simulink model "ClosedLoop_V5_2020b"  (R2020b)
settings: Solver=ode4  StartTime=0.0  StopTime=TMax  FixedStep=DT  MaxStep=DT  RelTol=1e-3  EnableMultiTasking=on
undefined symbols (not defined in the file or in its folder): CertificationSettings, Control, DiscIntNeverNeededParam, Drivetrain, OutList, P_InitAngle, RPM_Init, sigbuilder_block, SimConfig, strmatch
libraries: simulink x11, simulink_extras x6
(part 2 of 3)

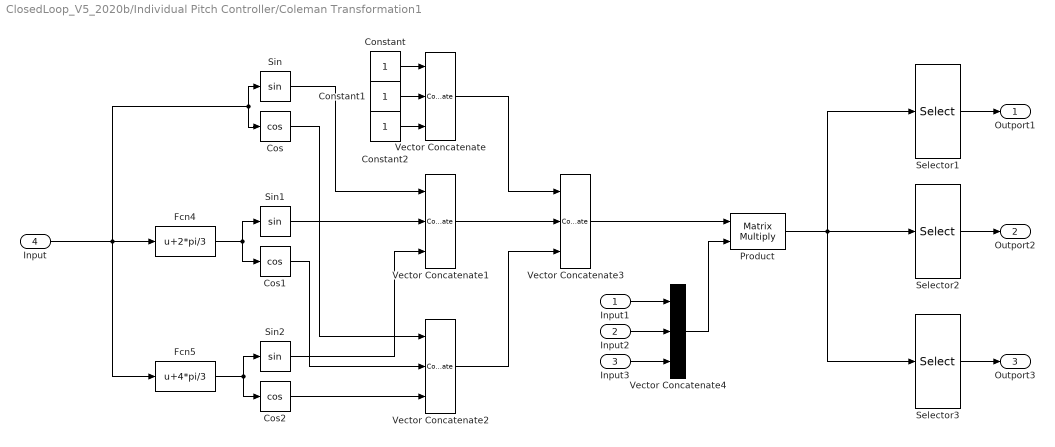
== system ClosedLoop_V5_2020b/Individual Pitch Controller/Coleman Transformation1 ==
  Input1 : Inport
  Input2 : Inport  Port=2
  Input3 : Inport  Port=3
  Input : Inport  Port=4
  Constant : Constant
  Constant1 : Constant
  Constant2 : Constant
  Cos : Trigonometry  Operator=cos
  Cos1 : Trigonometry  Operator=cos
  Cos2 : Trigonometry  Operator=cos
  Fcn4 : Fcn  Expr=u+2*pi/3
  Fcn5 : Fcn  Expr=u+4*pi/3
  Product : Product  Multiplication=Matrix(*)
  Selector1 : Selector  InputPortWidth=3  IndexOptions=Index vector (dialog)  Indices=[1]  OutputSizes=1
  Selector2 : Selector  InputPortWidth=3  IndexOptions=Index vector (dialog)  Indices=[2]  OutputSizes=1
  Selector3 : Selector  InputPortWidth=3  IndexOptions=Index vector (dialog)  Indices=[3]  OutputSizes=1
  Sin : Trigonometry
  Sin1 : Trigonometry
  Sin2 : Trigonometry
  Vector Concatenate{,1..2,4} (4 alike) : Concatenate  NumInputs=3
  Vector Concatenate3 : Concatenate  NumInputs=3  Mode=Multidimensional array  ConcatenateDimension=2
  Outport1 : Outport  VectorParamsAs1DForOutWhenUnconnected=off
  Outport2 : Outport  Port=2  VectorParamsAs1DForOutWhenUnconnected=off
  Outport3 : Outport  Port=3  VectorParamsAs1DForOutWhenUnconnected=off
  wires:
  Input3/1 -> Vector Concatenate4/3
  Input2/1 -> Vector Concatenate4/2
  Input1/1 -> Vector Concatenate4/1
  Constant2/1 -> Vector Concatenate/3
  Vector Concatenate3/1 -> Product/1
  Fcn4/1 -> Cos1/1, Sin1/1
  Vector Concatenate2/1 -> Vector Concatenate3/3
  Selector3/1 -> Outport3/1
  Selector2/1 -> Outport2/1
  Selector1/1 -> Outport1/1
  Vector Concatenate4/1 -> Product/2
  Vector Concatenate1/1 -> Vector Concatenate3/2
  Input/1 -> Cos/1, Sin/1, Fcn4/1, Fcn5/1
  Constant/1 -> Vector Concatenate/1
  Constant1/1 -> Vector Concatenate/2
  Sin2/1 -> Vector Concatenate1/3
  Cos1/1 -> Vector Concatenate2/2
  Cos/1 -> Vector Concatenate2/1
  Sin1/1 -> Vector Concatenate1/2
  Cos2/1 -> Vector Concatenate2/3
  Sin/1 -> Vector Concatenate1/1
  Product/1 -> Selector1/1, Selector2/1, Selector3/1
  Vector Concatenate/1 -> Vector Concatenate3/1
  Fcn5/1 -> Cos2/1, Sin2/1

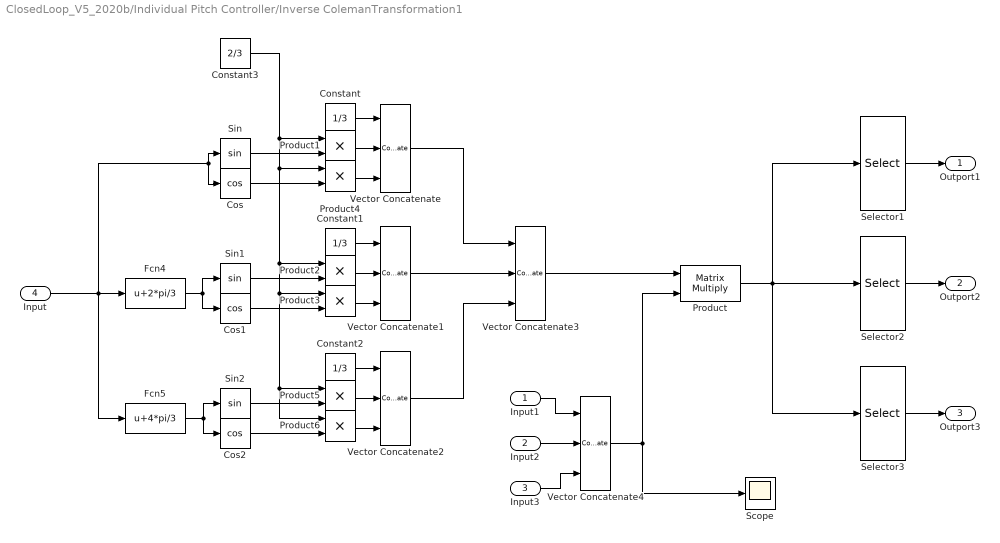
== system ClosedLoop_V5_2020b/Individual Pitch Controller/Inverse ColemanTransformation1 ==
  Input1 : Inport
  Input2 : Inport  Port=2
  Input3 : Inport  Port=3
  Input : Inport  Port=4
  Constant : Constant  Value=1/3
  Constant1 : Constant  Value=1/3
  Constant2 : Constant  Value=1/3
  Constant3 : Constant  Value=2/3
  Cos : Trigonometry  Operator=cos
  Cos1 : Trigonometry  Operator=cos
  Cos2 : Trigonometry  Operator=cos
  Fcn4 : Fcn  Expr=u+2*pi/3
  Fcn5 : Fcn  Expr=u+4*pi/3
  Product : Product  Multiplication=Matrix(*)
  Product{1..6} (6 alike) : Product
  Scope : Scope
  Selector1 : Selector  InputPortWidth=3  IndexOptions=Index vector (dialog)  Indices=[1]  OutputSizes=1
  Selector2 : Selector  InputPortWidth=3  IndexOptions=Index vector (dialog)  Indices=[2]  OutputSizes=1
  Selector3 : Selector  InputPortWidth=3  IndexOptions=Index vector (dialog)  Indices=[3]  OutputSizes=1
  Sin : Trigonometry
  Sin1 : Trigonometry
  Sin2 : Trigonometry
  Vector Concatenate : Concatenate  NumInputs=3  Mode=Multidimensional array
  Vector Concatenate1 : Concatenate  NumInputs=3  Mode=Multidimensional array
  Vector Concatenate2 : Concatenate  NumInputs=3  Mode=Multidimensional array
  Vector Concatenate3 : Concatenate  NumInputs=3  Mode=Multidimensional array  ConcatenateDimension=2
  Vector Concatenate4 : Concatenate  NumInputs=3
  Outport1 : Outport  VectorParamsAs1DForOutWhenUnconnected=off
  Outport2 : Outport  Port=2  VectorParamsAs1DForOutWhenUnconnected=off
  Outport3 : Outport  Port=3  VectorParamsAs1DForOutWhenUnconnected=off
  wires:
  Selector2/1 -> Outport2/1
  Selector3/1 -> Outport3/1
  Product/1 -> Selector1/1, Selector2/1, Selector3/1
  Selector1/1 -> Outport1/1
  Product2/1 -> Vector Concatenate1/2
  Product1/1 -> Vector Concatenate/2
  Constant/1 -> Vector Concatenate/1
  Vector Concatenate1/1 -> Vector Concatenate3/2
  Vector Concatenate2/1 -> Vector Concatenate3/3
  Vector Concatenate/1 -> Vector Concatenate3/1
  Vector Concatenate3/1 -> Product/1
  Input/1 -> Fcn4/1, Fcn5/1, Cos/1, Sin/1
  Product4/1 -> Vector Concatenate/3
  Sin1/1 -> Product2/2
  Constant1/1 -> Vector Concatenate1/1
  Product6/1 -> Vector Concatenate2/3
  Constant2/1 -> Vector Concatenate2/1
  Product3/1 -> Vector Concatenate1/3
  Sin/1 -> Product1/2
  Product5/1 -> Vector Concatenate2/2
  Input3/1 -> Vector Concatenate4/3
  Vector Concatenate4/1 -> Product/2, Scope/1
  Input1/1 -> Vector Concatenate4/1
  Input2/1 -> Vector Concatenate4/2
  Constant3/1 -> Product4/1, Product2/1, Product6/1, Product5/1, Product3/1, Product1/1
  Cos/1 -> Product4/2
  Cos1/1 -> Product3/2
  Sin2/1 -> Product5/2
  Cos2/1 -> Product6/2
  Fcn4/1 -> Sin1/1, Cos1/1
  Fcn5/1 -> Sin2/1, Cos2/1

== system ClosedLoop_V5_2020b/Individual Pitch Controller/Subsystem ==
  M_N2 : Inport
  Derivative : Derivative
  Gain : Gain  Gain=SimConfig.controller.IPC.K_P
  Gain1 : Gain  Gain=SimConfig.controller.IPC.K_D
  Gain3 : Gain  Gain=SimConfig.controller.IPC.K_I
  Integrator : Integrator
  Scope : Scope  NumInputPorts=5
  Scope1 : Scope  NumInputPorts=2
  Scope2 : Scope  NumInputPorts=2
  Scope3 : Scope  NumInputPorts=2
  Sum : Sum  Inputs=+++
  Input2 : Outport  VectorParamsAs1DForOutWhenUnconnected=off
  wires:
  Sum/1 -> Scope/4, Input2/1
  M_N2/1 -> Gain/1, Scope2/2, Gain3/1, Scope/5, Gain1/1  "E"
  Gain/1 -> Scope2/1, Scope/2, Sum/2  "P"
  Integrator/1 -> Scope1/2, Scope/3, Sum/3  "I"
  Derivative/1 -> Sum/1, Scope/1, Scope3/1  "D"
  Gain3/1 -> Integrator/1, Scope1/1
  Gain1/1 -> Derivative/1, Scope3/2

== system ClosedLoop_V5_2020b/Individual Pitch Controller/Subsystem1 ==
  M_N3 : Inport
  Derivative : Derivative
  Gain : Gain  Gain=SimConfig.controller.IPC.K_P
  Gain1 : Gain  Gain=SimConfig.controller.IPC.K_D
  Gain3 : Gain  Gain=SimConfig.controller.IPC.K_I
  Integrator : Integrator
  Scope : Scope  NumInputPorts=3
  Scope1 : Scope  NumInputPorts=2
  Scope2 : Scope  NumInputPorts=2
  Scope3 : Scope  NumInputPorts=2
  Sum : Sum  Inputs=+++
  Input3 : Outport  VectorParamsAs1DForOutWhenUnconnected=off
  wires:
  Derivative/1 -> Sum/1, Scope/1, Scope3/1  "D"
  Integrator/1 -> Scope/3, Sum/3, Scope1/2  "I"
  Gain/1 -> Sum/2, Scope/2, Scope2/1  "P"
  M_N3/1 -> Gain1/1, Scope2/2, Gain/1, Gain3/1
  Sum/1 -> Input3/1
  Gain3/1 -> Integrator/1, Scope1/1
  Gain1/1 -> Derivative/1, Scope3/2

== system ClosedLoop_V5_2020b/Notch filter TEF1/Notch filter TEF 1 ==
  u : Inport
  Damping : Constant  Value=0.06
  Frequ : Constant  Value=0.4*2*pi
  Gain : Gain  Gain=2
  Integrator : Integrator
  Integrator1 : Integrator
  Notch Gain : Constant  Value=10
  Product{,1..3} (4 alike) : Product
  Sum : Sum  Inputs=|++
  Sum1 : Sum  Inputs=++|
  Sum2 : Sum  Inputs=-+|
  Sum3 : Sum  Inputs=+-
  y : Outport
  wires:
  Product/1 -> Sum/2
  Sum/1 -> Sum3/2, y/1, Sum2/1
  Integrator/1 -> Product/1
  Integrator1/1 -> Product2/1
  Sum3/1 -> Integrator1/1
  Product1/1 -> Gain/1
  Product2/1 -> Sum1/2
  u/1 -> Sum/1, Product3/1, Sum3/1
  Product3/1 -> Sum2/2
  Sum2/1 -> Product1/2
  Sum1/1 -> Integrator/1
  Notch Gain/1 -> Product3/2
  Damping/1 -> Product1/1
  Frequ/1 -> Product/2, Product2/2
  Gain/1 -> Sum1/1

== system ClosedLoop_V5_2020b/Notch filter TEF1/Notch filter TEF 2 ==
  u : Inport
  Damping : Constant  Value=0.04
  Frequ : Constant  Value=0.6*2*pi
  Gain : Gain  Gain=2
  Integrator : Integrator
  Integrator1 : Integrator
  Notch Gain : Constant  Value=10
  Product{,1..3} (4 alike) : Product
  Sum : Sum  Inputs=|++
  Sum1 : Sum  Inputs=++|
  Sum2 : Sum  Inputs=-+|
  Sum3 : Sum  Inputs=+-
  y : Outport
  wires:
  Gain/1 -> Sum1/1
  Frequ/1 -> Product2/2, Product/2
  Damping/1 -> Product1/1
  Notch Gain/1 -> Product3/2
  Sum1/1 -> Integrator/1
  Sum2/1 -> Product1/2
  Product3/1 -> Sum2/2
  u/1 -> Sum3/1, Product3/1, Sum/1
  Product2/1 -> Sum1/2
  Product1/1 -> Gain/1
  Sum3/1 -> Integrator1/1
  Integrator1/1 -> Product2/1
  Integrator/1 -> Product/1
  Sum/1 -> Sum2/1, y/1, Sum3/2
  Product/1 -> Sum/2

== system ClosedLoop_V5_2020b/Notch filter TEF2/Notch filter TEF 1 ==
  u : Inport
  Damping : Constant  Value=0.06
  Frequ : Constant  Value=0.4*2*pi
  Gain : Gain  Gain=2
  Integrator : Integrator
  Integrator1 : Integrator
  Notch Gain : Constant  Value=10
  Product{,1..3} (4 alike) : Product
  Sum : Sum  Inputs=|++
  Sum1 : Sum  Inputs=++|
  Sum2 : Sum  Inputs=-+|
  Sum3 : Sum  Inputs=+-
  y : Outport
  wires:
  Gain/1 -> Sum1/1
  Frequ/1 -> Product2/2, Product/2
  Damping/1 -> Product1/1
  Notch Gain/1 -> Product3/2
  Sum1/1 -> Integrator/1
  Sum2/1 -> Product1/2
  Product3/1 -> Sum2/2
  u/1 -> Sum3/1, Product3/1, Sum/1
  Product2/1 -> Sum1/2
  Product1/1 -> Gain/1
  Sum3/1 -> Integrator1/1
  Integrator1/1 -> Product2/1
  Integrator/1 -> Product/1
  Sum/1 -> Sum2/1, y/1, Sum3/2
  Product/1 -> Sum/2

== system ClosedLoop_V5_2020b/Notch filter TEF2/Notch filter TEF 2 ==
  u : Inport
  Damping : Constant  Value=0.04
  Frequ : Constant  Value=0.6*2*pi
  Gain : Gain  Gain=2
  Integrator : Integrator
  Integrator1 : Integrator
  Notch Gain : Constant  Value=10
  Product{,1..3} (4 alike) : Product
  Sum : Sum  Inputs=|++
  Sum1 : Sum  Inputs=++|
  Sum2 : Sum  Inputs=-+|
  Sum3 : Sum  Inputs=+-
  y : Outport
  wires:
  Product/1 -> Sum/2
  Sum/1 -> Sum3/2, y/1, Sum2/1
  Integrator/1 -> Product/1
  Integrator1/1 -> Product2/1
  Sum3/1 -> Integrator1/1
  Product1/1 -> Gain/1
  Product2/1 -> Sum1/2
  u/1 -> Sum/1, Product3/1, Sum3/1
  Product3/1 -> Sum2/2
  Sum2/1 -> Product1/2
  Sum1/1 -> Integrator/1
  Notch Gain/1 -> Product3/2
  Damping/1 -> Product1/1
  Frequ/1 -> Product/2, Product2/2
  Gain/1 -> Sum1/1

== system ClosedLoop_V5_2020b/Notch filter TEF4/Notch filter TEF 1 ==
  u : Inport
  Damping : Constant  Value=0.06
  Frequ : Constant  Value=0.4*2*pi
  Gain : Gain  Gain=2
  Integrator : Integrator
  Integrator1 : Integrator
  Notch Gain : Constant  Value=10
  Product{,1..3} (4 alike) : Product
  Sum : Sum  Inputs=|++
  Sum1 : Sum  Inputs=++|
  Sum2 : Sum  Inputs=-+|
  Sum3 : Sum  Inputs=+-
  y : Outport
  wires:
  Gain/1 -> Sum1/1
  Frequ/1 -> Product2/2, Product/2
  Damping/1 -> Product1/1
  Notch Gain/1 -> Product3/2
  Sum1/1 -> Integrator/1
  Sum2/1 -> Product1/2
  Product3/1 -> Sum2/2
  u/1 -> Sum3/1, Product3/1, Sum/1
  Product2/1 -> Sum1/2
  Product1/1 -> Gain/1
  Sum3/1 -> Integrator1/1
  Integrator1/1 -> Product2/1
  Integrator/1 -> Product/1
  Sum/1 -> Sum2/1, y/1, Sum3/2
  Product/1 -> Sum/2

== system ClosedLoop_V5_2020b/Notch filter TEF4/Notch filter TEF 2 ==
  u : Inport
  Damping : Constant  Value=0.04
  Frequ : Constant  Value=0.6*2*pi
  Gain : Gain  Gain=2
  Integrator : Integrator
  Integrator1 : Integrator
  Notch Gain : Constant  Value=10
  Product{,1..3} (4 alike) : Product
  Sum : Sum  Inputs=|++
  Sum1 : Sum  Inputs=++|
  Sum2 : Sum  Inputs=-+|
  Sum3 : Sum  Inputs=+-
  y : Outport
  wires:
  Product/1 -> Sum/2
  Sum/1 -> Sum3/2, y/1, Sum2/1
  Integrator/1 -> Product/1
  Integrator1/1 -> Product2/1
  Sum3/1 -> Integrator1/1
  Product1/1 -> Gain/1
  Product2/1 -> Sum1/2
  u/1 -> Sum/1, Product3/1, Sum3/1
  Product3/1 -> Sum2/2
  Sum2/1 -> Product1/2
  Sum1/1 -> Integrator/1
  Notch Gain/1 -> Product3/2
  Damping/1 -> Product1/1
  Frequ/1 -> Product/2, Product2/2
  Gain/1 -> Sum1/1

== system ClosedLoop_V5_2020b/Notch filter TEF5/Notch filter TEF 1 ==
  u : Inport
  Damping : Constant  Value=0.06
  Frequ : Constant  Value=0.4*2*pi
  Gain : Gain  Gain=2
  Integrator : Integrator
  Integrator1 : Integrator
  Notch Gain : Constant  Value=10
  Product{,1..3} (4 alike) : Product
  Sum : Sum  Inputs=|++
  Sum1 : Sum  Inputs=++|
  Sum2 : Sum  Inputs=-+|
  Sum3 : Sum  Inputs=+-
  y : Outport
  wires:
  Gain/1 -> Sum1/1
  Frequ/1 -> Product2/2, Product/2
  Damping/1 -> Product1/1
  Notch Gain/1 -> Product3/2
  Sum1/1 -> Integrator/1
  Sum2/1 -> Product1/2
  Product3/1 -> Sum2/2
  u/1 -> Sum3/1, Product3/1, Sum/1
  Product2/1 -> Sum1/2
  Product1/1 -> Gain/1
  Sum3/1 -> Integrator1/1
  Integrator1/1 -> Product2/1
  Integrator/1 -> Product/1
  Sum/1 -> Sum2/1, y/1, Sum3/2
  Product/1 -> Sum/2

== system ClosedLoop_V5_2020b/Notch filter TEF5/Notch filter TEF 2 ==
  u : Inport
  Damping : Constant  Value=0.04
  Frequ : Constant  Value=0.6*2*pi
  Gain : Gain  Gain=2
  Integrator : Integrator
  Integrator1 : Integrator
  Notch Gain : Constant  Value=10
  Product{,1..3} (4 alike) : Product
  Sum : Sum  Inputs=|++
  Sum1 : Sum  Inputs=++|
  Sum2 : Sum  Inputs=-+|
  Sum3 : Sum  Inputs=+-
  y : Outport
  wires:
  Product/1 -> Sum/2
  Sum/1 -> Sum3/2, y/1, Sum2/1
  Integrator/1 -> Product/1
  Integrator1/1 -> Product2/1
  Sum3/1 -> Integrator1/1
  Product1/1 -> Gain/1
  Product2/1 -> Sum1/2
  u/1 -> Sum/1, Product3/1, Sum3/1
  Product3/1 -> Sum2/2
  Sum2/1 -> Product1/2
  Sum1/1 -> Integrator/1
  Notch Gain/1 -> Product3/2
  Damping/1 -> Product1/1
  Frequ/1 -> Product/2, Product2/2
  Gain/1 -> Sum1/1

== system ClosedLoop_V5_2020b/Notch filter TEF6/Notch filter TEF 1 ==
  u : Inport
  Damping : Constant  Value=0.06
  Frequ : Constant  Value=0.4*2*pi
  Gain : Gain  Gain=2
  Integrator : Integrator
  Integrator1 : Integrator
  Notch Gain : Constant  Value=10
  Product{,1..3} (4 alike) : Product
  Sum : Sum  Inputs=|++
  Sum1 : Sum  Inputs=++|
  Sum2 : Sum  Inputs=-+|
  Sum3 : Sum  Inputs=+-
  y : Outport
  wires:
  Gain/1 -> Sum1/1
  Frequ/1 -> Product2/2, Product/2
  Damping/1 -> Product1/1
  Notch Gain/1 -> Product3/2
  Sum1/1 -> Integrator/1
  Sum2/1 -> Product1/2
  Product3/1 -> Sum2/2
  u/1 -> Sum3/1, Product3/1, Sum/1
  Product2/1 -> Sum1/2
  Product1/1 -> Gain/1
  Sum3/1 -> Integrator1/1
  Integrator1/1 -> Product2/1
  Integrator/1 -> Product/1
  Sum/1 -> Sum2/1, y/1, Sum3/2
  Product/1 -> Sum/2

== system ClosedLoop_V5_2020b/Notch filter TEF6/Notch filter TEF 2 ==
  u : Inport
  Damping : Constant  Value=0.04
  Frequ : Constant  Value=0.6*2*pi
  Gain : Gain  Gain=2
  Integrator : Integrator
  Integrator1 : Integrator
  Notch Gain : Constant  Value=10
  Product{,1..3} (4 alike) : Product
  Sum : Sum  Inputs=|++
  Sum1 : Sum  Inputs=++|
  Sum2 : Sum  Inputs=-+|
  Sum3 : Sum  Inputs=+-
  y : Outport
  wires:
  Product/1 -> Sum/2
  Sum/1 -> Sum3/2, y/1, Sum2/1
  Integrator/1 -> Product/1
  Integrator1/1 -> Product2/1
  Sum3/1 -> Integrator1/1
  Product1/1 -> Gain/1
  Product2/1 -> Sum1/2
  u/1 -> Sum/1, Product3/1, Sum3/1
  Product3/1 -> Sum2/2
  Sum2/1 -> Product1/2
  Sum1/1 -> Integrator/1
  Notch Gain/1 -> Product3/2
  Damping/1 -> Product1/1
  Frequ/1 -> Product/2, Product2/2
  Gain/1 -> Sum1/1

== system ClosedLoop_V5_2020b/Notch filter Test/Notch filter 2 ==
  u : Inport
  gain : Inport  Port=2
  damping : Inport  Port=3
  frequency : Inport  Port=4
  Gain : Gain  Gain=2
  Integrator : Integrator
  Integrator1 : Integrator
  Product{,1..3} (4 alike) : Product
  Sum : Sum  Inputs=|++
  Sum1 : Sum  Inputs=++|
  Sum2 : Sum  Inputs=-+|
  Sum3 : Sum  Inputs=+-
  y : Outport
  wires:
  Gain/1 -> Sum1/1
  frequency/1 -> Product2/2, Product/2
  damping/1 -> Product1/1
  gain/1 -> Product3/2
  Sum1/1 -> Integrator/1
  Sum2/1 -> Product1/2
  Product3/1 -> Sum2/2
  u/1 -> Sum3/1, Product3/1, Sum/1
  Product2/1 -> Sum1/2
  Product1/1 -> Gain/1
  Sum3/1 -> Integrator1/1
  Integrator1/1 -> Product2/1
  Integrator/1 -> Product/1
  Sum/1 -> Sum2/1, y/1, Sum3/2
  Product/1 -> Sum/2

== system ClosedLoop_V5_2020b/Notch filter Test/Notch filter 3 ==
  u : Inport
  gain : Inport  Port=2
  damping : Inport  Port=3
  frequency : Inport  Port=4
  Gain : Gain  Gain=2
  Integrator : Integrator
  Integrator1 : Integrator
  Product{,1..3} (4 alike) : Product
  Sum : Sum  Inputs=|++
  Sum1 : Sum  Inputs=++|
  Sum2 : Sum  Inputs=-+|
  Sum3 : Sum  Inputs=+-
  y : Outport
  wires:
  Product/1 -> Sum/2
  Sum/1 -> Sum3/2, y/1, Sum2/1
  Integrator/1 -> Product/1
  Integrator1/1 -> Product2/1
  Sum3/1 -> Integrator1/1
  Product1/1 -> Gain/1
  Product2/1 -> Sum1/2
  u/1 -> Sum/1, Product3/1, Sum3/1
  Product3/1 -> Sum2/2
  Sum2/1 -> Product1/2
  Sum1/1 -> Integrator/1
  gain/1 -> Product3/2
  damping/1 -> Product1/1
  frequency/1 -> Product/2, Product2/2
  Gain/1 -> Sum1/1

== system ClosedLoop_V5_2020b/Notch filter Test/Notch filter neu ==
  u : Inport
  gain : Inport  Port=2
  damping : Inport  Port=3
  frequency : Inport  Port=4
  Gain : Gain  Gain=2
  Integrator : Integrator
  Integrator1 : Integrator
  Product{,1..3} (4 alike) : Product
  Sum : Sum  Inputs=|++
  Sum1 : Sum  Inputs=++|
  Sum2 : Sum  Inputs=-+|
  Sum3 : Sum  Inputs=+-
  y : Outport
  wires:
  Product/1 -> Sum/2
  Sum/1 -> Sum3/2, y/1, Sum2/1
  Integrator/1 -> Product/1
  Integrator1/1 -> Product2/1
  Sum3/1 -> Integrator1/1
  Product1/1 -> Gain/1
  Product2/1 -> Sum1/2
  u/1 -> Sum/1, Product3/1, Sum3/1
  Product3/1 -> Sum2/2
  Sum2/1 -> Product1/2
  Sum1/1 -> Integrator/1
  gain/1 -> Product3/2
  damping/1 -> Product1/1
  frequency/1 -> Product/2, Product2/2
  Gain/1 -> Sum1/1

== system ClosedLoop_V5_2020b/Notch filter Test/Subsystem ==
  u : Inport
  Notch filter TEF 1 : Subsystem
  Notch filter TEF 2 : Subsystem
  Scope : Scope  NumInputPorts=4
  Sum : Sum  Inputs=|++
  y : Outport
  wires:
  u/1 -> Notch filter TEF 2/1(u), Scope/4, Notch filter TEF 1/1(u)
  Notch filter TEF 1/1(y) -> Scope/2, Sum/1
  Notch filter TEF 2/1(y) -> Sum/2, Scope/3
  Sum/1 -> Scope/1, y/1

== system ClosedLoop_V5_2020b/Plot aerodynamic Data/Plot Angle of Attack ==
  OutData : Inport
  Scope1 : Scope  NumInputPorts=9
  Scope10 : Scope  NumInputPorts=3
  Scope12 : Scope  NumInputPorts=3
  Scope16 : Scope  NumInputPorts=3
  extract Angle of Attack : Fcn  Expr=u(strmatch('B1N1Alpha',OutList))
  extract Angle of Attack1 : Fcn  Expr=u(strmatch('B1N2Alpha',OutList))
  extract Angle of Attack2 : Fcn  Expr=u(strmatch('B1N3Alpha',OutList))
  extract Angle of Attack3 : Fcn  Expr=u(strmatch('B1N4Alpha',OutList))
  extract Angle of Attack4 : Fcn  Expr=u(strmatch('B1N5Alpha',OutList))
  extract Angle of Attack5 : Fcn  Expr=u(strmatch('B1N6Alpha',OutList))
  extract Angle of Attack6 : Fcn  Expr=u(strmatch('B1N7Alpha',OutList))
  extract Angle of Attack7 : Fcn  Expr=u(strmatch('B1N8Alpha',OutList))
  extract Angle of Attack8 : Fcn  Expr=u(strmatch('B1N9Alpha',OutList))
  wires:
  OutData/1 -> extract Angle of Attack8/1, extract Angle of Attack7/1, extract Angle of Attack6/1, extract Angle of Attack5/1, extract Angle of Attack4/1, extract Angle of Attack3/1, extract Angle of Attack2/1, extract Angle of Attack1/1, extract Angle of Attack/1
  extract Angle of Attack7/1 -> Scope1/8, Scope16/2  "Angle of Attack (deg)"
  extract Angle of Attack4/1 -> Scope1/5, Scope12/2  "Angle of Attack (deg)"
  extract Angle of Attack8/1 -> Scope1/9, Scope16/3  "Angle of Attack (deg)"
  extract Angle of Attack6/1 -> Scope1/7, Scope16/1  "Angle of Attack (deg)"
  extract Angle of Attack1/1 -> Scope1/2, Scope10/2  "Angle of Attack (deg)"
  extract Angle of Attack3/1 -> Scope1/4, Scope12/1  "Angle of Attack (deg)"
  extract Angle of Attack5/1 -> Scope1/6, Scope12/3  "Angle of Attack (deg)"
  extract Angle of Attack/1 -> Scope1/1, Scope10/1  "Angle of Attack (deg)"
  extract Angle of Attack2/1 -> Scope1/3, Scope10/3  "Angle of Attack (deg)"

== system ClosedLoop_V5_2020b/Plot aerodynamic Data/Plot Cd ==
  OutData : Inport
  Scope1 : Scope  NumInputPorts=9
  extract Cd : Fcn  Expr=u(strmatch('B1N1Cd',OutList))
  extract Cd1 : Fcn  Expr=u(strmatch('B1N2Cd',OutList))
  extract Cd2 : Fcn  Expr=u(strmatch('B1N3Cd',OutList))
  extract Cd3 : Fcn  Expr=u(strmatch('B1N4Cd',OutList))
  extract Cd4 : Fcn  Expr=u(strmatch('B1N5Cd',OutList))
  extract Cd5 : Fcn  Expr=u(strmatch('B1N6Cd',OutList))
  extract Cd6 : Fcn  Expr=u(strmatch('B1N7Cd',OutList))
  extract Cd7 : Fcn  Expr=u(strmatch('B1N8Cd',OutList))
  extract Cd8 : Fcn  Expr=u(strmatch('B1N9Cd',OutList))
  wires:
  OutData/1 -> extract Cd4/1, extract Cd5/1, extract Cd6/1, extract Cd8/1, extract Cd7/1, extract Cd3/1, extract Cd2/1, extract Cd1/1, extract Cd/1
  extract Cd/1 -> Scope1/1  "Cd"
  extract Cd1/1 -> Scope1/2  "Cd"
  extract Cd3/1 -> Scope1/4  "Cd"
  extract Cd2/1 -> Scope1/3  "Cd"
  extract Cd4/1 -> Scope1/5  "Cd"
  extract Cd5/1 -> Scope1/6  "Cd"
  extract Cd6/1 -> Scope1/7  "Cd"
  extract Cd7/1 -> Scope1/8  "Cd"
  extract Cd8/1 -> Scope1/9  "Cd"

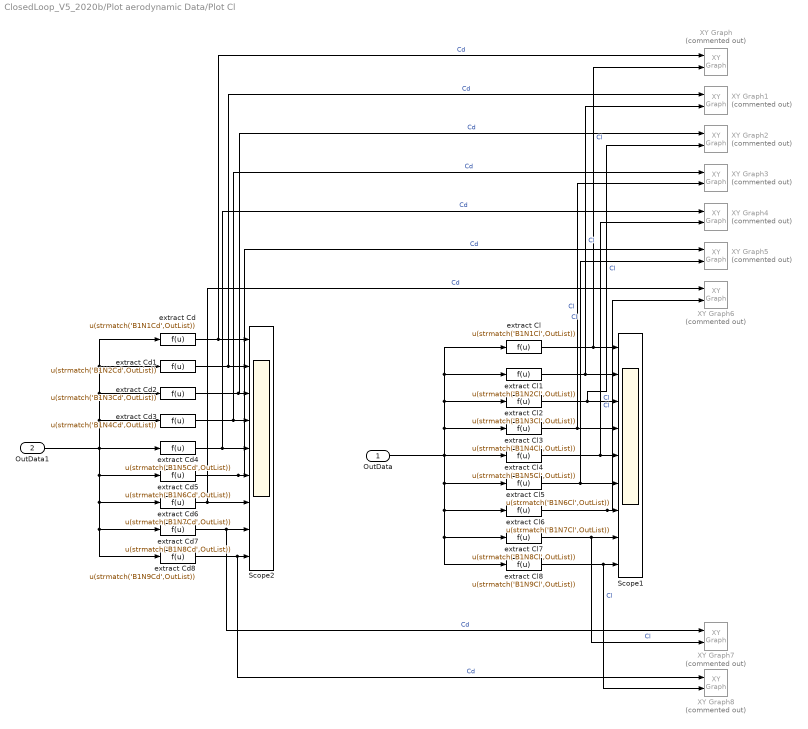
== system ClosedLoop_V5_2020b/Plot aerodynamic Data/Plot Cl ==
  OutData : Inport
  OutData1 : Inport  Port=2
  Scope1 : Scope  NumInputPorts=9
  Scope2 : Scope  NumInputPorts=9
  XY Graph{,1..8} (9 alike) : simulink/Sinks/XY Graph  Commented=on  xmin=-1  xmax=1  ymin=-1  ymax=1  st=-1
  extract Cd : Fcn  Expr=u(strmatch('B1N1Cd',OutList))
  extract Cd1 : Fcn  Expr=u(strmatch('B1N2Cd',OutList))
  extract Cd2 : Fcn  Expr=u(strmatch('B1N3Cd',OutList))
  extract Cd3 : Fcn  Expr=u(strmatch('B1N4Cd',OutList))
  extract Cd4 : Fcn  Expr=u(strmatch('B1N5Cd',OutList))
  extract Cd5 : Fcn  Expr=u(strmatch('B1N6Cd',OutList))
  extract Cd6 : Fcn  Expr=u(strmatch('B1N7Cd',OutList))
  extract Cd7 : Fcn  Expr=u(strmatch('B1N8Cd',OutList))
  extract Cd8 : Fcn  Expr=u(strmatch('B1N9Cd',OutList))
  extract Cl : Fcn  Expr=u(strmatch('B1N1Cl',OutList))
  extract Cl1 : Fcn  Expr=u(strmatch('B1N2Cl',OutList))
  extract Cl2 : Fcn  Expr=u(strmatch('B1N3Cl',OutList))
  extract Cl3 : Fcn  Expr=u(strmatch('B1N4Cl',OutList))
  extract Cl4 : Fcn  Expr=u(strmatch('B1N5Cl',OutList))
  extract Cl5 : Fcn  Expr=u(strmatch('B1N6Cl',OutList))
  extract Cl6 : Fcn  Expr=u(strmatch('B1N7Cl',OutList))
  extract Cl7 : Fcn  Expr=u(strmatch('B1N8Cl',OutList))
  extract Cl8 : Fcn  Expr=u(strmatch('B1N9Cl',OutList))
  wires:
  OutData/1 -> extract Cl/1, extract Cl1/1, extract Cl2/1, extract Cl3/1, extract Cl4/1, extract Cl5/1, extract Cl6/1, extract Cl8/1, extract Cl7/1
  extract Cl/1 -> XY Graph/2, Scope1/1  "Cl"
  extract Cl1/1 -> XY Graph1/2, Scope1/2  "Cl"
  extract Cl2/1 -> XY Graph2/2, Scope1/3  "Cl"
  extract Cl3/1 -> XY Graph3/2, Scope1/4  "Cl"
  extract Cl4/1 -> XY Graph4/2, Scope1/5  "Cl"
  extract Cl5/1 -> XY Graph5/2, Scope1/6  "Cl"
  extract Cl6/1 -> XY Graph6/2, Scope1/7  "Cl"
  extract Cl7/1 -> XY Graph7/2, Scope1/8  "Cl"
  extract Cl8/1 -> XY Graph8/2, Scope1/9  "Cl"
  extract Cd2/1 -> XY Graph2/1, Scope2/3  "Cd"
  extract Cd8/1 -> XY Graph8/1, Scope2/9  "Cd"
  extract Cd4/1 -> XY Graph4/1, Scope2/5  "Cd"
  extract Cd3/1 -> XY Graph3/1, Scope2/4  "Cd"
  extract Cd/1 -> XY Graph/1, Scope2/1  "Cd"
  OutData1/1 -> extract Cd4/1, extract Cd5/1, extract Cd6/1, extract Cd8/1, extract Cd7/1, extract Cd3/1, extract Cd2/1, extract Cd1/1, extract Cd/1
  extract Cd1/1 -> XY Graph1/1, Scope2/2  "Cd"
  extract Cd7/1 -> XY Graph7/1, Scope2/8  "Cd"
  extract Cd5/1 -> XY Graph5/1, Scope2/6  "Cd"
  extract Cd6/1 -> Scope2/7, XY Graph6/1  "Cd"

== system ClosedLoop_V5_2020b/Plot aerodynamic Data/Plot Pitch+Twist Angle ==
  OutData : Inport
  Add{,1..8} (9 alike) : Sum  Inputs=+-
  Scope1 : Scope  NumInputPorts=9
  Scope2 : Scope  NumInputPorts=9
  extract BldPitch1 (deg) : Fcn  Expr=u(strmatch('BldPitch1',OutList))
  extract Pitch+Twist angle : Fcn  Expr=u(strmatch('B1N1Theta',OutList))
  extract Pitch+Twist angle1 : Fcn  Expr=u(strmatch('B1N2Theta',OutList))
  extract Pitch+Twist angle2 : Fcn  Expr=u(strmatch('B1N3Theta',OutList))
  extract Pitch+Twist angle3 : Fcn  Expr=u(strmatch('B1N4Theta',OutList))
  extract Pitch+Twist angle4 : Fcn  Expr=u(strmatch('B1N5Theta',OutList))
  extract Pitch+Twist angle5 : Fcn  Expr=u(strmatch('B1N6Theta',OutList))
  extract Pitch+Twist angle6 : Fcn  Expr=u(strmatch('B1N7Theta',OutList))
  extract Pitch+Twist angle7 : Fcn  Expr=u(strmatch('B1N8Theta',OutList))
  extract Pitch+Twist angle8 : Fcn  Expr=u(strmatch('B1N9Theta',OutList))
  wires:
  extract Pitch+Twist angle/1 -> Add/1, Scope1/1  "Pitch+Twist angle (deg)"
  OutData/1 -> extract Pitch+Twist angle/1, extract Pitch+Twist angle1/1, extract Pitch+Twist angle2/1, extract Pitch+Twist angle3/1, extract Pitch+Twist angle4/1, extract Pitch+Twist angle5/1, extract Pitch+Twist angle6/1, extract BldPitch1 (deg)/1, extract Pitch+Twist angle8/1, extract Pitch+Twist angle7/1
  extract Pitch+Twist angle1/1 -> Add1/1, Scope1/2  "Pitch+Twist angle (deg)"
  extract Pitch+Twist angle2/1 -> Add2/1, Scope1/3  "Pitch+Twist angle (deg)"
  extract Pitch+Twist angle3/1 -> Add3/1, Scope1/4  "Pitch+Twist angle (deg)"
  extract Pitch+Twist angle4/1 -> Add4/1, Scope1/5  "Pitch+Twist angle (deg)"
  extract Pitch+Twist angle5/1 -> Add5/1, Scope1/6  "Pitch+Twist angle (deg)"
  extract Pitch+Twist angle6/1 -> Add6/1, Scope1/7  "Pitch+Twist angle (deg)"
  extract Pitch+Twist angle7/1 -> Add7/1, Scope1/8  "Pitch+Twist angle (deg)"
  extract Pitch+Twist angle8/1 -> Add8/1, Scope1/9  "Pitch+Twist angle (deg)"
  extract BldPitch1 (deg)/1 -> Add8/2, Add7/2, Add6/2, Add5/2, Add4/2, Add3/2, Add2/2, Add1/2, Add/2  "BldPitch1"
  Add/1 -> Scope2/1
  Add1/1 -> Scope2/2
  Add2/1 -> Scope2/3
  Add3/1 -> Scope2/4
  Add4/1 -> Scope2/5
  Add5/1 -> Scope2/6
  Add6/1 -> Scope2/7
  Add7/1 -> Scope2/8
  Add8/1 -> Scope2/9

== system ClosedLoop_V5_2020b/Plot aerodynamic Data/Plot Relative Wind Speed ==
  OutData1 : Inport
  Scope : Scope  NumInputPorts=9
  "extract Relative Wind Speed (m/s) at Blade 1, Node 1" : Fcn  Expr=u(strmatch('B1N1VRel',OutList))
  "extract Relative Wind Speed (m/s) at Blade 1, Node 2" : Fcn  Expr=u(strmatch('B1N2VRel',OutList))
  "extract Relative Wind Speed (m/s) at Blade 1, Node 3" : Fcn  Expr=u(strmatch('B1N3VRel',OutList))
  "extract Relative Wind Speed (m/s) at Blade 1, Node 4" : Fcn  Expr=u(strmatch('B1N4VRel',OutList))
  "extract Relative Wind Speed (m/s) at Blade 1, Node 5" : Fcn  Expr=u(strmatch('B1N5VRel',OutList))
  "extract Relative Wind Speed (m/s) at Blade 1, Node 6" : Fcn  Expr=u(strmatch('B1N6VRel',OutList))
  "extract Relative Wind Speed (m/s) at Blade 1, Node 7" : Fcn  Expr=u(strmatch('B1N7VRel',OutList))
  "extract Relative Wind Speed (m/s) at Blade 1, Node 8" : Fcn  Expr=u(strmatch('B1N8VRel',OutList))
  "extract Relative Wind Speed (m/s) at Blade 1, Node 9" : Fcn  Expr=u(strmatch('B1N9VRel',OutList))
  wires:
  OutData1/1 -> "extract Relative Wind Speed (m/s) at Blade 1, Node 9"/1, "extract Relative Wind Speed (m/s) at Blade 1, Node 8"/1, "extract Relative Wind Speed (m/s) at Blade 1, Node 7"/1, "extract Relative Wind Speed (m/s) at Blade 1, Node 6"/1, "extract Relative Wind Speed (m/s) at Blade 1, Node 5"/1, "extract Relative Wind Speed (m/s) at Blade 1, Node 4"/1, "extract Relative Wind Speed (m/s) at Blade 1, Node 3"/1, "extract Relative Wind Speed (m/s) at Blade 1, Node 2"/1, "extract Relative Wind Speed (m/s) at Blade 1, Node 1"/1
  "extract Relative Wind Speed (m/s) at Blade 1, Node 6"/1 -> Scope/6  "Relative Wind Speed (m/s) at Blade 1, Node 6"
  "extract Relative Wind Speed (m/s) at Blade 1, Node 7"/1 -> Scope/7  "Relative Wind Speed (m/s) at Blade 1, Node 7"
  "extract Relative Wind Speed (m/s) at Blade 1, Node 5"/1 -> Scope/5  "Relative Wind Speed (m/s) at Blade 1, Node 5"
  "extract Relative Wind Speed (m/s) at Blade 1, Node 9"/1 -> Scope/9  "Relative Wind Speed (m/s) at Blade 1, Node 9"
  "extract Relative Wind Speed (m/s) at Blade 1, Node 2"/1 -> Scope/2  "Relative Wind Speed (m/s) at Blade 1, Node 2"
  "extract Relative Wind Speed (m/s) at Blade 1, Node 1"/1 -> Scope/1  "Relative Wind Speed (m/s) at Blade 1, Node 1"
  "extract Relative Wind Speed (m/s) at Blade 1, Node 8"/1 -> Scope/8  "Relative Wind Speed (m/s) at Blade 1, Node 8"
  "extract Relative Wind Speed (m/s) at Blade 1, Node 4"/1 -> Scope/4  "Relative Wind Speed (m/s) at Blade 1, Node 4"
  "extract Relative Wind Speed (m/s) at Blade 1, Node 3"/1 -> Scope/3  "Relative Wind Speed (m/s) at Blade 1, Node 3"

== system ClosedLoop_V5_2020b/Plot aerodynamic Data/Plot Reynolds number ==
  note: B1N1Re      Reynolds number (in millions) at Blade 1, Node 1
      | B1N2Re      Reynolds number (in millions) at Blade 1, Node 2
      | B1N3Re      Reynolds number (in millions) at Blade 1, Node 3
      | B1N4Re      Reynolds number (in millions) at Blade 1, Node 4
      | B1N5Re      Reynolds number (in millions) at Blade 1, Node 5
      | B1N6Re      Reynolds number (in millions) at Blade 1, Node 6
      | B1N7Re      Reynolds number (in millions) at Blade 1, Node 7
      | B1N8Re      Reynolds number (in millions) at Blade 1, Node 8
      | B1N9Re      Reynolds number (in millions) at Blade 1, Node 9
  OutData1 : Inport
  Scope : Scope  NumInputPorts=9
  "extract Reynolds number (in millions) at Blade 1, Node 1" : Fcn  Expr=u(strmatch('B1N1Re',OutList))
  "extract Reynolds number (in millions) at Blade 1, Node 2" : Fcn  Expr=u(strmatch('B1N2Re',OutList))
  "extract Reynolds number (in millions) at Blade 1, Node 3" : Fcn  Expr=u(strmatch('B1N3Re',OutList))
  "extract Reynolds number (in millions) at Blade 1, Node 4" : Fcn  Expr=u(strmatch('B1N4Re',OutList))
  "extract Reynolds number (in millions) at Blade 1, Node 5" : Fcn  Expr=u(strmatch('B1N5Re',OutList))
  "extract Reynolds number (in millions) at Blade 1, Node 6" : Fcn  Expr=u(strmatch('B1N6Re',OutList))
  "extract Reynolds number (in millions) at Blade 1, Node 7" : Fcn  Expr=u(strmatch('B1N7Re',OutList))
  "extract Reynolds number (in millions) at Blade 1, Node 8" : Fcn  Expr=u(strmatch('B1N8Re',OutList))
  "extract Reynolds number (in millions) at Blade 1, Node 9" : Fcn  Expr=u(strmatch('B1N9Re',OutList))
  wires:
  OutData1/1 -> "extract Reynolds number (in millions) at Blade 1, Node 9"/1, "extract Reynolds number (in millions) at Blade 1, Node 8"/1, "extract Reynolds number (in millions) at Blade 1, Node 7"/1, "extract Reynolds number (in millions) at Blade 1, Node 6"/1, "extract Reynolds number (in millions) at Blade 1, Node 5"/1, "extract Reynolds number (in millions) at Blade 1, Node 4"/1, "extract Reynolds number (in millions) at Blade 1, Node 3"/1, "extract Reynolds number (in millions) at Blade 1, Node 2"/1, "extract Reynolds number (in millions) at Blade 1, Node 1"/1
  "extract Reynolds number (in millions) at Blade 1, Node 8"/1 -> Scope/8  "Reynolds number (in millions) at Blade 1, Node 8"
  "extract Reynolds number (in millions) at Blade 1, Node 3"/1 -> Scope/3  "Reynolds number (in millions) at Blade 1, Node 3"
  "extract Reynolds number (in millions) at Blade 1, Node 5"/1 -> Scope/5  "Reynolds number (in millions) at Blade 1, Node 5"
  "extract Reynolds number (in millions) at Blade 1, Node 7"/1 -> Scope/7  "Reynolds number (in millions) at Blade 1, Node 7"
  "extract Reynolds number (in millions) at Blade 1, Node 1"/1 -> Scope/1  "Reynolds number (in millions) at Blade 1, Node 1"
  "extract Reynolds number (in millions) at Blade 1, Node 6"/1 -> Scope/6  "Reynolds number (in millions) at Blade 1, Node 6"
  "extract Reynolds number (in millions) at Blade 1, Node 4"/1 -> Scope/4  "Reynolds number (in millions) at Blade 1, Node 4"
  "extract Reynolds number (in millions) at Blade 1, Node 9"/1 -> Scope/9  "Reynolds number (in millions) at Blade 1, Node 9"
  "extract Reynolds number (in millions) at Blade 1, Node 2"/1 -> Scope/2  "Reynolds number (in millions) at Blade 1, Node 2"

== system ClosedLoop_V5_2020b/Plot aerodynamic Data/Plot Rotor Data ==
  note: RtAeroFxh   Total rotor aerodynamic load (force in x direction) the hub coordinate system N
      | RtAeroFyh   Total rotor aerodynamic load (force in y direction) the hub coordinate system N
      | RtAeroFzh   Total rotor aerodynamic load (force in z direction) the hub coordinate system N
      | RtAeroMxh   Total rotor aerodynamic load (moment in x direction) the hub coordinate system Nm
      | RtAeroMyh   Total rotor aerodynamic load (moment in y direction) the hub coordinate system Nm
      | RtAeroMzh   Total rotor aerodynamic load (moment in z direction) the hub coordinate system Nm
      | RtAeroPwr   Rotor aerodynamic power W
      | RtAeroCp    Rotor aerodynamic power coefficient
      | RtAeroCq    Rotor aerodynamic torque coefficient
      | RtAeroCt    Rotor aerodynamic thrust coefficient
  OutData : Inport
  Scope : Scope  NumInputPorts=3
  Scope1 : Scope  NumInputPorts=3
  Scope{2..5} (4 alike) : Scope
  extract Rotor aerodynamic power W : Fcn  Expr=u(strmatch('RtAeroPwr',OutList))
  extract Rotor aerodynamic power coefficient : Fcn  Expr=u(strmatch('RtAeroCp',OutList))
  extract Rotor aerodynamic thrust coefficient : Fcn  Expr=u(strmatch('RtAeroCt',OutList))
  extract Rotor aerodynamic torque coefficient : Fcn  Expr=u(strmatch('RtAeroCp',OutList))
  extract Total rotor aerodynamic load (force in x direction) hub coordinate system (N) : Fcn  Expr=u(strmatch('RtAeroFxh',OutList))
  extract Total rotor aerodynamic load (force in y direction) hub coordinate system (N) : Fcn  Expr=u(strmatch('RtAeroFyh',OutList))
  extract Total rotor aerodynamic load (force in z direction) hub coordinate system (N) : Fcn  Expr=u(strmatch('RtAeroFzh',OutList))
  extract Total rotor aerodynamic load (moment in x direction) the hub coordinate system Nm : Fcn  Expr=u(strmatch('RtAeroMxh',OutList))
  extract Total rotor aerodynamic load (moment in y direction) the hub coordinate system Nm : Fcn  Expr=u(strmatch('RtAeroMyh',OutList))
  extract Total rotor aerodynamic load (moment in z direction) the hub coordinate system Nm : Fcn  Expr=u(strmatch('RtAeroMzh',OutList))
  wires:
  extract Total rotor aerodynamic load (force in x direction) hub coordinate system (N)/1 -> Scope/1  "Total rotor aerodynamic load (force in x direction) hub coordinate system (N)"
  OutData/1 -> extract Rotor aerodynamic thrust coefficient/1, extract Rotor aerodynamic torque coefficient/1, extract Rotor aerodynamic power coefficient/1, extract Rotor aerodynamic power W/1, extract Total rotor aerodynamic load (moment in z direction) the hub coordinate system Nm/1, extract Total rotor aerodynamic load (moment in y direction) the hub coordinate system Nm/1, extract Total rotor aerodynamic load (force in z direction) hub coordinate system (N)/1, extract Total rotor aerodynamic load (force in y direction) hub coordinate system (N)/1, extract Total rotor aerodynamic load (force in x direction) hub coordinate system (N)/1, extract Total rotor aerodynamic load (moment in x direction) the hub coordinate system Nm/1
  extract Total rotor aerodynamic load (force in y direction) hub coordinate system (N)/1 -> Scope/2  "Total rotor aerodynamic load (force in y direction) hub coordinate system (N)"
  extract Total rotor aerodynamic load (force in z direction) hub coordinate system (N)/1 -> Scope/3  "Total rotor aerodynamic load (force in z direction) hub coordinate system (N)"
  extract Total rotor aerodynamic load (moment in x direction) the hub coordinate system Nm/1 -> Scope1/1  "Total rotor aerodynamic load (moment in x direction) the hub coordinate system Nm"
  extract Total rotor aerodynamic load (moment in y direction) the hub coordinate system Nm/1 -> Scope1/2  "Total rotor aerodynamic load (moment in y direction) the hub coordinate system Nm"
  extract Total rotor aerodynamic load (moment in z direction) the hub coordinate system Nm/1 -> Scope1/3  "Total rotor aerodynamic load (moment in z direction) the hub coordinate system Nm"
  extract Rotor aerodynamic power W/1 -> Scope2/1  "Rotor aerodynamic power W"
  extract Rotor aerodynamic power coefficient/1 -> Scope3/1  "Rotor aerodynamic power coefficient"
  extract Rotor aerodynamic torque coefficient/1 -> Scope4/1  "Rotor aerodynamic torque coefficient"
  extract Rotor aerodynamic thrust coefficient/1 -> Scope5/1  "Rotor aerodynamic thrust coefficient"

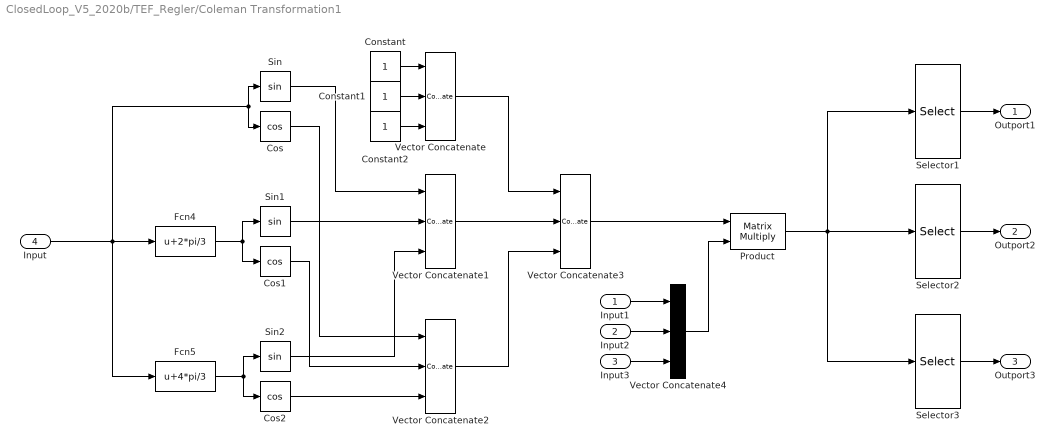
== system ClosedLoop_V5_2020b/TEF_Regler/Coleman Transformation1 ==
  Input1 : Inport
  Input2 : Inport  Port=2
  Input3 : Inport  Port=3
  Input : Inport  Port=4
  Constant : Constant
  Constant1 : Constant
  Constant2 : Constant
  Cos : Trigonometry  Operator=cos
  Cos1 : Trigonometry  Operator=cos
  Cos2 : Trigonometry  Operator=cos
  Fcn4 : Fcn  Expr=u+2*pi/3
  Fcn5 : Fcn  Expr=u+4*pi/3
  Product : Product  Multiplication=Matrix(*)
  Selector1 : Selector  InputPortWidth=3  IndexOptions=Index vector (dialog)  Indices=[1]  OutputSizes=1
  Selector2 : Selector  InputPortWidth=3  IndexOptions=Index vector (dialog)  Indices=[2]  OutputSizes=1
  Selector3 : Selector  InputPortWidth=3  IndexOptions=Index vector (dialog)  Indices=[3]  OutputSizes=1
  Sin : Trigonometry
  Sin1 : Trigonometry
  Sin2 : Trigonometry
  Vector Concatenate{,1..2,4} (4 alike) : Concatenate  NumInputs=3
  Vector Concatenate3 : Concatenate  NumInputs=3  Mode=Multidimensional array  ConcatenateDimension=2
  Outport1 : Outport  VectorParamsAs1DForOutWhenUnconnected=off
  Outport2 : Outport  Port=2  VectorParamsAs1DForOutWhenUnconnected=off
  Outport3 : Outport  Port=3  VectorParamsAs1DForOutWhenUnconnected=off
  wires:
  Input3/1 -> Vector Concatenate4/3
  Input2/1 -> Vector Concatenate4/2
  Input1/1 -> Vector Concatenate4/1
  Constant2/1 -> Vector Concatenate/3
  Vector Concatenate3/1 -> Product/1
  Fcn4/1 -> Cos1/1, Sin1/1
  Vector Concatenate2/1 -> Vector Concatenate3/3
  Selector3/1 -> Outport3/1
  Selector2/1 -> Outport2/1
  Selector1/1 -> Outport1/1
  Vector Concatenate4/1 -> Product/2
  Vector Concatenate1/1 -> Vector Concatenate3/2
  Input/1 -> Cos/1, Sin/1, Fcn4/1, Fcn5/1
  Constant/1 -> Vector Concatenate/1
  Constant1/1 -> Vector Concatenate/2
  Sin2/1 -> Vector Concatenate1/3
  Cos1/1 -> Vector Concatenate2/2
  Cos/1 -> Vector Concatenate2/1
  Sin1/1 -> Vector Concatenate1/2
  Cos2/1 -> Vector Concatenate2/3
  Sin/1 -> Vector Concatenate1/1
  Product/1 -> Selector1/1, Selector2/1, Selector3/1
  Vector Concatenate/1 -> Vector Concatenate3/1
  Fcn5/1 -> Cos2/1, Sin2/1

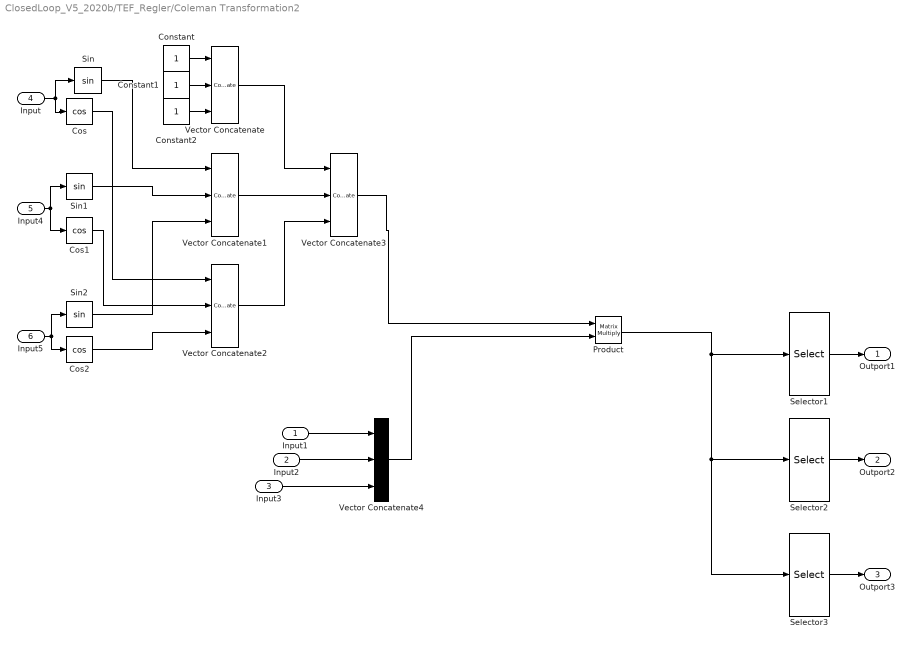
== system ClosedLoop_V5_2020b/TEF_Regler/Coleman Transformation2 ==
  Input1 : Inport
  Input2 : Inport  Port=2
  Input3 : Inport  Port=3
  Input : Inport  Port=4
  Input4 : Inport  Port=5
  Input5 : Inport  Port=6
  Constant : Constant
  Constant1 : Constant
  Constant2 : Constant
  Cos : Trigonometry  Operator=cos
  Cos1 : Trigonometry  Operator=cos
  Cos2 : Trigonometry  Operator=cos
  Product : Product  Multiplication=Matrix(*)
  Selector1 : Selector  InputPortWidth=3  IndexOptions=Index vector (dialog)  Indices=[1]  OutputSizes=1
  Selector2 : Selector  InputPortWidth=3  IndexOptions=Index vector (dialog)  Indices=[2]  OutputSizes=1
  Selector3 : Selector  InputPortWidth=3  IndexOptions=Index vector (dialog)  Indices=[3]  OutputSizes=1
  Sin : Trigonometry
  Sin1 : Trigonometry
  Sin2 : Trigonometry
  Vector Concatenate{,1..2,4} (4 alike) : Concatenate  NumInputs=3
  Vector Concatenate3 : Concatenate  NumInputs=3  Mode=Multidimensional array  ConcatenateDimension=2
  Outport1 : Outport  VectorParamsAs1DForOutWhenUnconnected=off
  Outport2 : Outport  Port=2  VectorParamsAs1DForOutWhenUnconnected=off
  Outport3 : Outport  Port=3  VectorParamsAs1DForOutWhenUnconnected=off
  wires:
  Input3/1 -> Vector Concatenate4/3
  Input2/1 -> Vector Concatenate4/2
  Input1/1 -> Vector Concatenate4/1
  Constant2/1 -> Vector Concatenate/3
  Vector Concatenate3/1 -> Product/1
  Input4/1 -> Sin1/1, Cos1/1
  Vector Concatenate2/1 -> Vector Concatenate3/3
  Selector3/1 -> Outport3/1
  Selector2/1 -> Outport2/1
  Selector1/1 -> Outport1/1
  Vector Concatenate4/1 -> Product/2
  Vector Concatenate1/1 -> Vector Concatenate3/2
  Input5/1 -> Sin2/1, Cos2/1
  Constant/1 -> Vector Concatenate/1
  Constant1/1 -> Vector Concatenate/2
  Sin2/1 -> Vector Concatenate1/3
  Cos1/1 -> Vector Concatenate2/2
  Cos/1 -> Vector Concatenate2/1
  Sin1/1 -> Vector Concatenate1/2
  Cos2/1 -> Vector Concatenate2/3
  Sin/1 -> Vector Concatenate1/1
  Input/1 -> Sin/1, Cos/1
  Product/1 -> Selector1/1, Selector2/1, Selector3/1
  Vector Concatenate/1 -> Vector Concatenate3/1

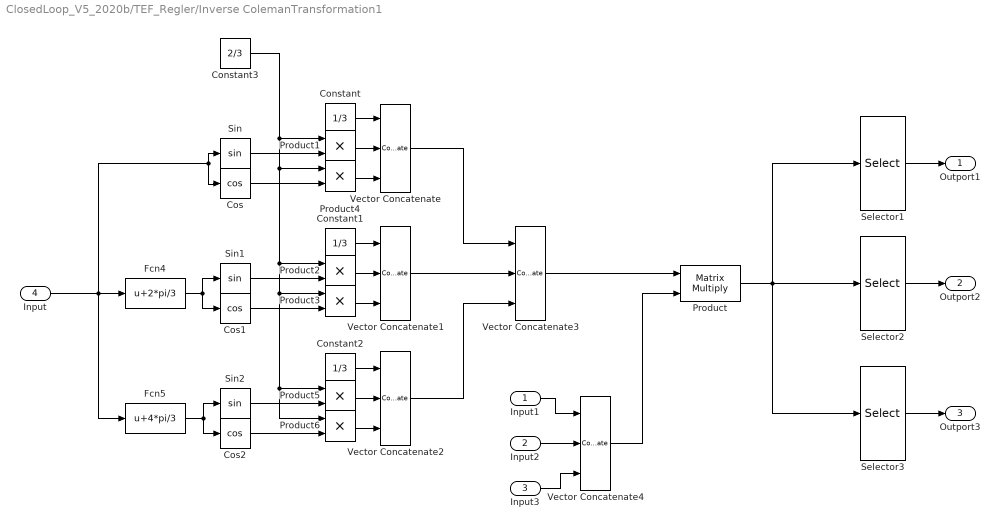
== system ClosedLoop_V5_2020b/TEF_Regler/Inverse ColemanTransformation1 ==
  Input1 : Inport
  Input2 : Inport  Port=2
  Input3 : Inport  Port=3
  Input : Inport  Port=4
  Constant : Constant  Value=1/3
  Constant1 : Constant  Value=1/3
  Constant2 : Constant  Value=1/3
  Constant3 : Constant  Value=2/3
  Cos : Trigonometry  Operator=cos
  Cos1 : Trigonometry  Operator=cos
  Cos2 : Trigonometry  Operator=cos
  Fcn4 : Fcn  Expr=u+2*pi/3
  Fcn5 : Fcn  Expr=u+4*pi/3
  Product : Product  Multiplication=Matrix(*)
  Product{1..6} (6 alike) : Product
  Selector1 : Selector  InputPortWidth=3  IndexOptions=Index vector (dialog)  Indices=[1]  OutputSizes=1
  Selector2 : Selector  InputPortWidth=3  IndexOptions=Index vector (dialog)  Indices=[2]  OutputSizes=1
  Selector3 : Selector  InputPortWidth=3  IndexOptions=Index vector (dialog)  Indices=[3]  OutputSizes=1
  Sin : Trigonometry
  Sin1 : Trigonometry
  Sin2 : Trigonometry
  Vector Concatenate : Concatenate  NumInputs=3  Mode=Multidimensional array
  Vector Concatenate1 : Concatenate  NumInputs=3  Mode=Multidimensional array
  Vector Concatenate2 : Concatenate  NumInputs=3  Mode=Multidimensional array
  Vector Concatenate3 : Concatenate  NumInputs=3  Mode=Multidimensional array  ConcatenateDimension=2
  Vector Concatenate4 : Concatenate  NumInputs=3
  Outport1 : Outport  VectorParamsAs1DForOutWhenUnconnected=off
  Outport2 : Outport  Port=2  VectorParamsAs1DForOutWhenUnconnected=off
  Outport3 : Outport  Port=3  VectorParamsAs1DForOutWhenUnconnected=off
  wires:
  Selector2/1 -> Outport2/1
  Selector3/1 -> Outport3/1
  Product/1 -> Selector1/1, Selector2/1, Selector3/1
  Selector1/1 -> Outport1/1
  Product2/1 -> Vector Concatenate1/2
  Product1/1 -> Vector Concatenate/2
  Constant/1 -> Vector Concatenate/1
  Vector Concatenate1/1 -> Vector Concatenate3/2
  Vector Concatenate2/1 -> Vector Concatenate3/3
  Vector Concatenate/1 -> Vector Concatenate3/1
  Vector Concatenate3/1 -> Product/1
  Input/1 -> Fcn4/1, Fcn5/1, Cos/1, Sin/1
  Product4/1 -> Vector Concatenate/3
  Sin1/1 -> Product2/2
  Constant1/1 -> Vector Concatenate1/1
  Product6/1 -> Vector Concatenate2/3
  Constant2/1 -> Vector Concatenate2/1
  Product3/1 -> Vector Concatenate1/3
  Sin/1 -> Product1/2
  Product5/1 -> Vector Concatenate2/2
  Input3/1 -> Vector Concatenate4/3
  Vector Concatenate4/1 -> Product/2
  Input1/1 -> Vector Concatenate4/1
  Input2/1 -> Vector Concatenate4/2
  Constant3/1 -> Product4/1, Product2/1, Product6/1, Product5/1, Product3/1, Product1/1
  Cos/1 -> Product4/2
  Cos1/1 -> Product3/2
  Sin2/1 -> Product5/2
  Cos2/1 -> Product6/2
  Fcn4/1 -> Sin1/1, Cos1/1
  Fcn5/1 -> Sin2/1, Cos2/1

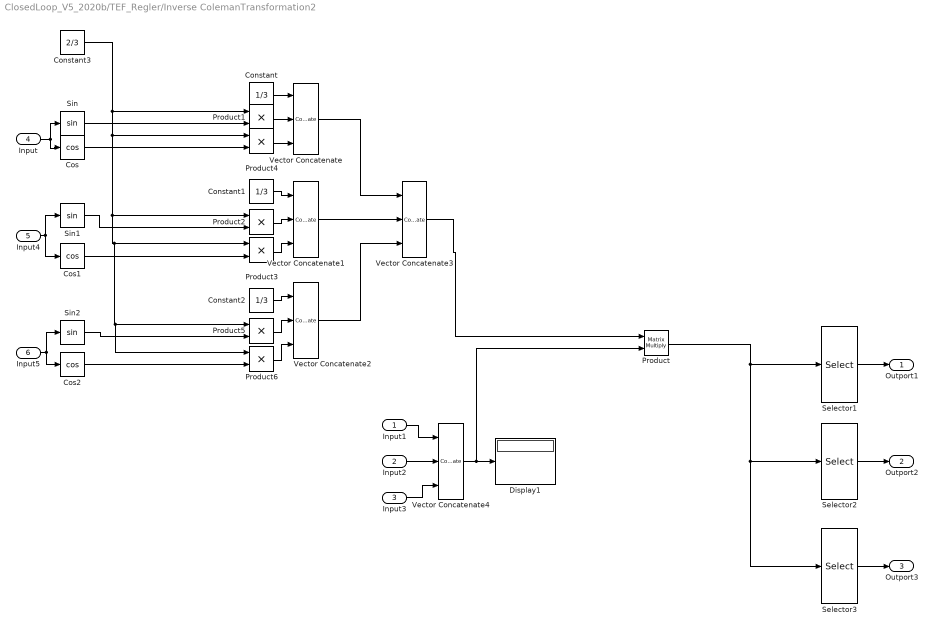
== system ClosedLoop_V5_2020b/TEF_Regler/Inverse ColemanTransformation2 ==
  Input1 : Inport
  Input2 : Inport  Port=2
  Input3 : Inport  Port=3
  Input : Inport  Port=4
  Input4 : Inport  Port=5
  Input5 : Inport  Port=6
  Constant : Constant  Value=1/3
  Constant1 : Constant  Value=1/3
  Constant2 : Constant  Value=1/3
  Constant3 : Constant  Value=2/3
  Cos : Trigonometry  Operator=cos
  Cos1 : Trigonometry  Operator=cos
  Cos2 : Trigonometry  Operator=cos
  Display1 : Display
  Product : Product  Multiplication=Matrix(*)
  Product{1..6} (6 alike) : Product
  Selector1 : Selector  InputPortWidth=3  IndexOptions=Index vector (dialog)  Indices=[1]  OutputSizes=1
  Selector2 : Selector  InputPortWidth=3  IndexOptions=Index vector (dialog)  Indices=[2]  OutputSizes=1
  Selector3 : Selector  InputPortWidth=3  IndexOptions=Index vector (dialog)  Indices=[3]  OutputSizes=1
  Sin : Trigonometry
  Sin1 : Trigonometry
  Sin2 : Trigonometry
  Vector Concatenate{,1..2,4} (4 alike) : Concatenate  NumInputs=3  Mode=Multidimensional array
  Vector Concatenate3 : Concatenate  NumInputs=3  Mode=Multidimensional array  ConcatenateDimension=2
  Outport1 : Outport  VectorParamsAs1DForOutWhenUnconnected=off
  Outport2 : Outport  Port=2  VectorParamsAs1DForOutWhenUnconnected=off
  Outport3 : Outport  Port=3  VectorParamsAs1DForOutWhenUnconnected=off
  wires:
  Selector2/1 -> Outport2/1
  Selector3/1 -> Outport3/1
  Product/1 -> Selector1/1, Selector2/1, Selector3/1
  Selector1/1 -> Outport1/1
  Input4/1 -> Sin1/1, Cos1/1
  Product2/1 -> Vector Concatenate1/2
  Product1/1 -> Vector Concatenate/2
  Constant/1 -> Vector Concatenate/1
  Vector Concatenate1/1 -> Vector Concatenate3/2
  Vector Concatenate2/1 -> Vector Concatenate3/3
  Input/1 -> Cos/1, Sin/1
  Vector Concatenate/1 -> Vector Concatenate3/1
  Vector Concatenate3/1 -> Product/1
  Input5/1 -> Sin2/1, Cos2/1
  Product4/1 -> Vector Concatenate/3
  Sin1/1 -> Product2/2
  Constant1/1 -> Vector Concatenate1/1
  Product6/1 -> Vector Concatenate2/3
  Constant2/1 -> Vector Concatenate2/1
  Product3/1 -> Vector Concatenate1/3
  Sin/1 -> Product1/2
  Product5/1 -> Vector Concatenate2/2
  Input3/1 -> Vector Concatenate4/3
  Vector Concatenate4/1 -> Display1/1, Product/2
  Input1/1 -> Vector Concatenate4/1
  Input2/1 -> Vector Concatenate4/2
  Constant3/1 -> Product1/1, Product4/1, Product2/1, Product3/1, Product5/1, Product6/1
  Cos/1 -> Product4/2
  Cos1/1 -> Product3/2
  Sin2/1 -> Product5/2
  Cos2/1 -> Product6/2

== system ClosedLoop_V5_2020b/TEF_Regler/Subsystem ==
  In1 : Inport
  Derivative : Derivative
  Gain : Gain  Gain=SimConfig.controller.TEF.K_P
  Gain1 : Gain  Gain=SimConfig.controller.TEF.K_I
  Gain2 : Gain  Gain=SimConfig.controller.TEF.K_D
  Integrator : Integrator
  Scope : Scope  NumInputPorts=2
  Scope1 : Scope  NumInputPorts=2
  Scope2 : Scope  NumInputPorts=4
  Sum : Sum  Inputs=+++
  Input2 : Outport  VectorParamsAs1DForOutWhenUnconnected=off
  wires:
  Sum/1 -> Scope2/4, Input2/1
  Integrator/1 -> Gain1/1  "I"
  Derivative/1 -> Gain2/1
  In1/1 -> Scope/1, Gain/1, Scope1/2, Integrator/1, Derivative/1
  Gain/1 -> Scope/2, Scope2/2, Sum/2  "P"
  Gain1/1 -> Scope1/1, Scope2/3, Sum/3  "I"
  Gain2/1 -> Scope2/1, Sum/1  "D"

== system ClosedLoop_V5_2020b/TEF_Regler/Subsystem1 ==
  In1 : Inport
  Derivative : Derivative
  Gain : Gain  Gain=SimConfig.controller.TEF.K_P
  Gain1 : Gain  Gain=SimConfig.controller.TEF.K_I
  Gain2 : Gain  Gain=SimConfig.controller.TEF.K_D
  Integrator : Integrator
  Sum : Sum  Inputs=+++
  Input3 : Outport  VectorParamsAs1DForOutWhenUnconnected=off
  wires:
  Gain2/1 -> Sum/1
  Gain1/1 -> Sum/3
  Gain/1 -> Sum/2
  In1/1 -> Derivative/1, Integrator/1, Gain/1
  Derivative/1 -> Gain2/1
  Integrator/1 -> Gain1/1
  Sum/1 -> Input3/1

== system ClosedLoop_V5_2020b/TEF_Regler/Subsystem2 ==
  In1 : Inport
  Derivative : Derivative
  Gain : Gain  Gain=SimConfig.controller.TEF.K_P
  Gain1 : Gain  Gain=SimConfig.controller.TEF.K_I
  Gain2 : Gain  Gain=SimConfig.controller.TEF.K_D
  Integrator : Integrator
  Scope : Scope  NumInputPorts=2
  Scope1 : Scope  NumInputPorts=2
  Scope2 : Scope  NumInputPorts=5
  Sum : Sum  Inputs=+++
  M_N2 : Outport  VectorParamsAs1DForOutWhenUnconnected=off
  wires:
  Gain2/1 -> Scope2/1, Sum/1  "D"
  Gain1/1 -> Sum/3, Scope2/3, Scope1/1
  Gain/1 -> Sum/2, Scope2/2, Scope/2  "P"
  In1/1 -> Derivative/1, Integrator/1, Scope1/2, Gain/1, Scope/1, Scope2/5
  Derivative/1 -> Gain2/1
  Integrator/1 -> Gain1/1  "I"
  Sum/1 -> M_N2/1, Scope2/4

== system ClosedLoop_V5_2020b/TEF_Regler/Subsystem3 ==
  In1 : Inport
  Derivative : Derivative
  Gain : Gain  Gain=SimConfig.controller.TEF.K_P
  Gain1 : Gain  Gain=SimConfig.controller.TEF.K_I
  Gain2 : Gain  Gain=SimConfig.controller.TEF.K_D
  Integrator : Integrator
  Sum : Sum  Inputs=+++
  M_N3 : Outport  VectorParamsAs1DForOutWhenUnconnected=off
  wires:
  Sum/1 -> M_N3/1
  Integrator/1 -> Gain1/1
  Derivative/1 -> Gain2/1
  In1/1 -> Gain/1, Integrator/1, Derivative/1
  Gain/1 -> Sum/2
  Gain1/1 -> Sum/3
  Gain2/1 -> Sum/1
